simulink model "Hw03_P1_Spec1"  (R2024a)
settings: Solver=VariableStepAuto  StartTime=0.0  StopTime=10.0  RelTol=1e-3
settings Model: Creator=bojack  LastModifiedBy=bojack
settings OptimizationCC: ReuseModelBlockBuffer=off
settings RTWCC: GPUComputeCapability=3.5

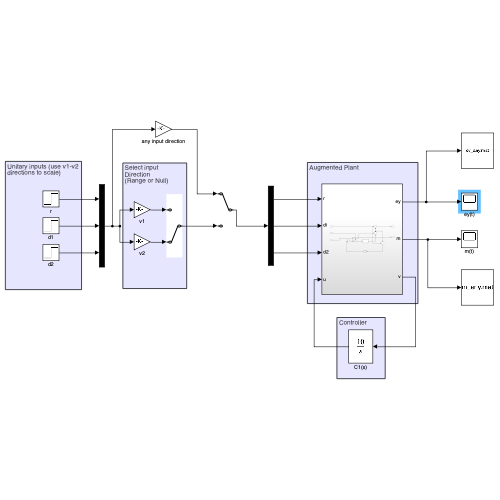
[thumbnail: Simulink's stored preview of the top-level diagram]
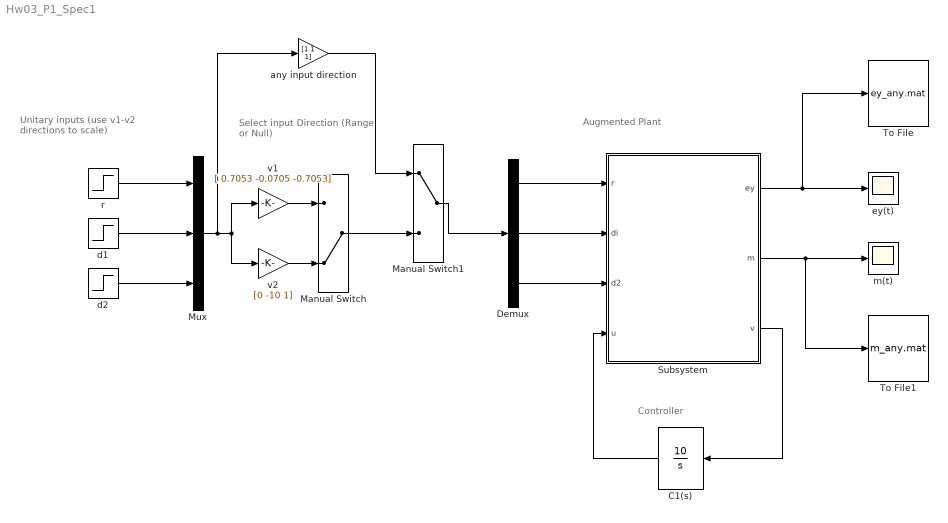
== system Hw03_P1_Spec1 ==
  note: Controller
  note: Augmented Plant
  note: Unitary inputs (use v1-v2
      | directions to scale)
  note: Select input
      | Direction
      | (Range or Null)
  C1(s) : TransferFcn  Numerator=[10]  Denominator=[1 0]
  Demux : Demux  Outputs=3
  Manual Switch : ManualSwitch  CurrentSetting=0
  Manual Switch1 : ManualSwitch
  Mux : Mux  Inputs=3
  Subsystem : Subsystem
  To File : ToFile  Filename=ey_any.mat  SaveFormat=Timeseries
  To File1 : ToFile  Filename=m_any.mat  SaveFormat=Timeseries
  any input direction : Gain  Gain=[1 1 1]
  d1 : Step  Time=0  SampleTime=0
  d2 : Step  Time=0  SampleTime=0
  ey(t) : Scope
  m(t) : Scope
  r : Step  Time=0  SampleTime=0
  v1 : Gain  Gain=[ 0.7053 -0.0705 -0.7053]
  v2 : Gain  Gain=[0 -10 1]
  wires:
  C1(s)/1 -> Subsystem/4(u)
  Subsystem/1(ey) -> To File/1, ey(t)/1
  Subsystem/2(m) -> To File1/1, m(t)/1
  Subsystem/3(v) -> C1(s)/1
  d1/1 -> Mux/2
  Demux/1 -> Subsystem/1(r)
  Demux/2 -> Subsystem/2(di)
  Demux/3 -> Subsystem/3(d2)
  d2/1 -> Mux/3
  r/1 -> Mux/1
  v1/1 -> Manual Switch/1
  v2/1 -> Manual Switch/2
  Mux/1 -> v1/1, v2/1, any input direction/1
  Manual Switch/1 -> Manual Switch1/2
  Manual Switch1/1 -> Demux/1
  any input direction/1 -> Manual Switch1/1

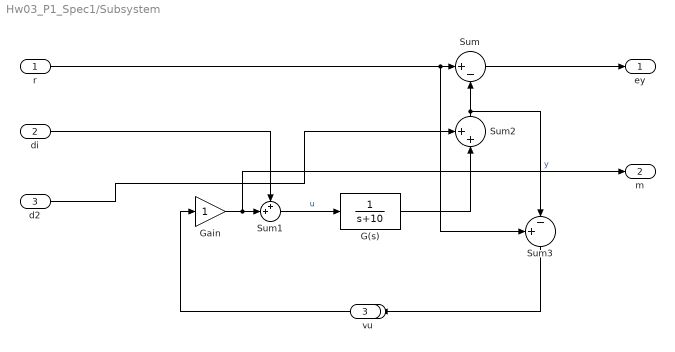
== system Hw03_P1_Spec1/Subsystem ==
  r : Inport
  di : Inport  Port=2
  d2 : Inport  Port=3
  u : Inport  Port=4
  G(s) : TransferFcn  Denominator=[1 10]
  Gain : Gain
  Sum : Sum  Inputs=|+-
  Sum1 : Sum  Inputs=++|
  Sum2 : Sum  Inputs=++|
  Sum3 : Sum  Inputs=+-|
  ey : Outport
  m : Outport  Port=2
  v : Outport  Port=3
  wires:
  Sum3/1 -> v/1
  di/1 -> Sum1/1
  d2/1 -> Sum2/1
  Gain/1 -> m/1, Sum1/2
  Sum/1 -> ey/1
  G(s)/1 -> Sum2/2
  r/1 -> Sum3/1, Sum/1
  Sum2/1 -> Sum3/2, Sum/2  "y"
  u/1 -> Gain/1
  Sum1/1 -> G(s)/1  "u"
